simulink model "test3"  (R2023a)
settings: Solver=VariableStepAuto  StartTime=0.0  StopTime=10.0  RelTol=1e-3
settings Model: Creator=BQ  LastModifiedBy=BQ

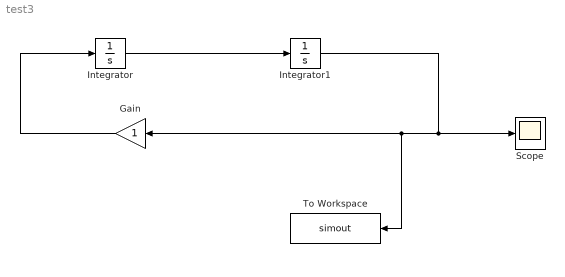
== system test3 ==
  Gain : Gain
  Integrator : Integrator
  Integrator1 : Integrator  InitialCondition=1
  Scope : Scope
  To Workspace : ToWorkspace  VariableName=simout  SaveFormat=Timeseries  SampleTime=-1
  wires:
  Integrator/1 -> Integrator1/1
  Gain/1 -> Integrator/1
  Integrator1/1 -> To Workspace/1, Gain/1, Scope/1
